simulink model "PhaseEquivalentFOCModel"  (R2020b)
settings: Solver=VariableStepAuto  StartTime=0.0  StopTime=10.0  RelTol=1e-3
libraries: ee_lib x7, nesl_utility x7, mcbcontrolslib x2, eeTransforms x1, eePmsmCurrentController x1, powerlib_meascontrol x1, eeVelocityController x1
settings Model: Creator=trgre  LastModifiedBy=trgre

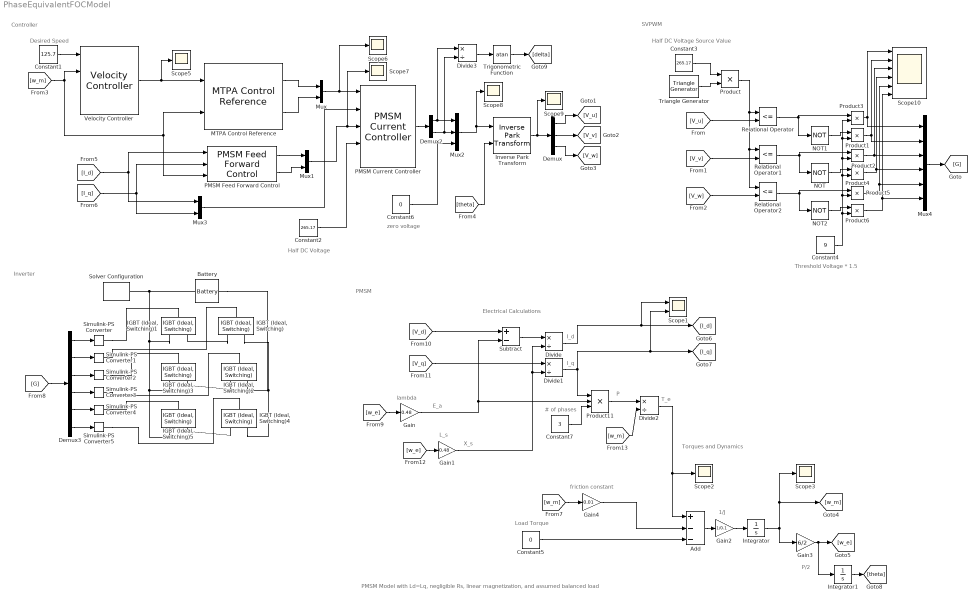
== system PhaseEquivalentFOCModel ==
  note: Load Torque
  note: friction constant
  note: Inverter
  note: PMSM
  note: P/2
  note: 1/J
  note: lambda
  note: Torques and Dynamics
  note: Electrical Calculations
  note: T_e
  note: # of phases
  note: P
  note: PMSM Model with Ld=Lq, negligible Rs, linear magnetization, and assumed balanced load
  note: I_q
  note: I_d
  note: X_s
  note: L_s
  note: E_a
  note: Controller
  note: SVPWM
  note: Desired Speed
  note: Half DC Voltage
  note: zero voltage
  note: Threshold Voltage * 1.5
  note: Half DC Voltage Source Value
  Add : Sum  Inputs=+--
  Battery : ee_lib/Sources/Battery  Vnom=530.35 V  prm_dir=1  R1_dis=2 Ohm  R1_ch=2 Ohm  R1=0.01 Ohm  prm_AH=1  AH=50 hr*A  V1=11.5 V  AH1=25 hr*A  prm_R2=1  R2=2000 Ohm  prm_dyn=1  Rp1=0.005 Ohm  tau1=30 s  Rp2=0.005 Ohm  tau2=30 s  Rp3=0.005 Ohm  tau3=30 s  Rp4=0.005 Ohm  tau4=30 s  Rp5=0.005 Ohm  tau5=30 s  prm_fade=1  N_fade=100  AH_fade=45 hr*A  R1_fade=2.02 Ohm  R1_ch_fade=2.02 Ohm  V1_fade=10.35 V  i_specify=off  i_priority=None  i=0 A  i_nominal_specify=off  i_nominal_unit=A  i_nominal_value=1  v_specify=off  v_priority=None  v=0 V  v_nominal_specify=off  v_nominal_unit=V  v_nominal_value=1  charge_specify=off  charge_priority=High  charge=50 hr*A  charge_nominal_specify=off  charge_nominal_unit=hr*A  charge_nominal_value=1  num_cycles_specify=off  num_cycles_priority=High  num_cycles=0  num_cycles_nominal_specify=off  num_cycles_nominal_unit=1  num_cycles_nominal_value=1  thermal_mass=30000 J/K  Tmeas=298.15 K  Vnom_T2=12 V  R1_T2=2.2 Ohm  R1_T2_dis=2.2 Ohm  R1_T2_ch=2.2 Ohm  V1_T2=11.4 V  R2_T2=2200 Ohm  Rp1_T2=0.005 Ohm  tau1_T2=30 s  Rp2_T2=0.005 Ohm  tau2_T2=30 s  Rp3_T2=0.005 Ohm  tau3_T2=30 s  Rp4_T2=0.005 Ohm  tau4_T2=30 s  Rp5_T2=0.005 Ohm  tau5_T2=30 s  Tmeas2=273.15 K  temperature_specify=off  temperature_priority=High  temperature=298.15 K  temperature_nominal_specify=off  temperature_nominal_unit=K  temperature_nominal_value=1
  Constant1 : Constant  Value=125.7
  Constant2 : Constant  Value=265.17
  Constant3 : Constant  Value=265.17
  Constant4 : Constant  Value=9
  Constant5 : Constant  Value=0
  Constant6 : Constant  Value=0
  Constant7 : Constant  Value=3
  Demux : Demux  Outputs=3
  Demux2 : Demux  Outputs=2
  Demux3 : Demux  Outputs=6
  Divide{,1..3} (4 alike) : Product  Inputs=*/
  Gain : Gain  Gain=0.48
  Gain1 : Gain  Gain=0.48
  Gain2 : Gain  Gain=1/0.1
  Gain3 : Gain  Gain=6/2
  Gain4 : Gain  Gain=0.01
  IGBT (Ideal, Switching){,1..5} (6 alike) : ee_lib/Semiconductors & Converters/IGBT (Ideal, Switching)  Vf=0.8 V  Ron=0.001 Ohm  Goff=1e-5 1/Ohm  Vth=6 V  diode_param=2  diode_Vf=0.8 V  diode_Ron=0.001 Ohm  diode_Goff=1e-5 1/Ohm  diode_C=50e-9 F  diode_iRM=-235 A  diode_iF=300 A  diode_idot=-50 A/us  diode_trr_param=1  diode_trr_factor=3  diode_trr=15 us  diode_Qrr=1500 s*uA  thermal_loss_option=ee.enum.converters.thermalLossOption.constantvalues  Von_data=[0, .1, .6, .8, 1, 1.3, 1.6, 2, 2.4; 0, .1, .7, 1, 1.2, 1.5, 1.9, 2.4, 2.8] V  Eon_data=[0, .0024, .024, .12, .2, .48, 1.04, 2.16, 3.24; 0, .003, .03, .15, .25, .6, 1.3, 2.7, 4.05] * 1e-3 J  Eoff_data=[0, .0007, .0066, .033, .066, .17, .33, .83, 1.5; 0, .001, .01, .05, .1, .25, .5, 1.2, 2.2] * 1e-3 J  Tj=[298.15, 398.15] K  Iout_data=[0, .1, 1, 5, 10, 20, 40, 70, 100] A  Eon_scalar=22.86e-3 J  Eoff_scalar=17.14e-3 J  Voff=300 V  Iout_scalar=600 A  diodeModelType=ee.enum.converters.diodeModelType.pwl  diode_IfMat=[.07, .12, .19, 1.75, 4.24, 7.32, 11.2; .16, .3, .72, 2.14, 4.02, 6.35, 9.12] A  diode_TjVec=[25, 125] degC  diode_VfVec=[.5, .7, .9, 1.3, 1.7, 2.1, 2.5] V  thermal_network_parameterization=ee.enum.thermalNetworkTopology.external  Rth=[.08, .5] K/W  Rth_Foster=[.08, .14, .22, .16] K/W  thermal_mass_parameterization=ee.enum.thermalNetwork.timeconstant  thermal_mass=[.01, .5] J/K  thermal_mass_Foster=[.001, .005, .05, .5] J/K  thermal_time_constant=[.001, .2] s  thermal_time_constant_Foster=[7e-05, .0007, .01, .08] s  thermal_mass_initial_temperatures=[25, 25] degC  junction_thermal_mass=0.01 J/K  Tau=1e-4 s  vT_specify=off  vT_priority=None  vT=0 V  vT_nominal_specify=off  vT_nominal_unit=V  vT_nominal_value=1  Qj_specify=off  Qj_priority=None  Qj=0 W  Qj_nominal_specify=off  Qj_nominal_unit=W  Qj_nominal_value=1  junction_temperature_specify=off  junction_temperature_priority=None  junction_temperature=25 degC  junction_temperature_nominal_specify=off  junction_temperature_nominal_unit=degC  junction_temperature_nominal_value=1
  Integrator : Integrator  InitialCondition=125.7
  Integrator1 : Integrator
  Inverse Park Transform : eeTransforms/Inverse Park Transform  AxisAlignment=Q-axis  PowerInvariant=off
  MTPA Control Reference : mcbcontrolslib/MTPA Control Reference  LabelModeActiveChoice=Surface PMSM  VariantSelect=Surface PMSM  polePairs=3  Rs=0.36  Ld=0.00137  Lq=0.4e-3  FluxPM=0.48  I_sat=7.1  V_dc=24  Units=SI Units  N_base=1200  I_base=19.3  T_base=1  N_base_disp=3182
      settings: SourceProductBaseCode=MT
  Mux : Mux  Inputs=2
  Mux1 : Mux  Inputs=2
  Mux2 : Mux  Inputs=3
  Mux3 : Mux  Inputs=2
  Mux4 : Mux  Inputs=6
  NOT : Logic  Operator=NOT  IconShape=distinctive  AllPortsSameDT=off  OutDataTypeStr=boolean
  NOT1 : Logic  Operator=NOT  IconShape=distinctive  AllPortsSameDT=off  OutDataTypeStr=boolean
  NOT2 : Logic  Operator=NOT  IconShape=distinctive  AllPortsSameDT=off  OutDataTypeStr=boolean
  PMSM Current Controller : eePmsmCurrentController/PMSM Current Controller  Kp_id=1  Ki_id=100  Kaw_id=1  Kp_iq=1  Ki_iq=100  Kaw_iq=1  Ts=-1  Tsd=0.001  AxisPrio=Q-axis  ActZC=off  ActFF=on
      settings: SourceProductBaseCode=PS
  PMSM Feed Forward Control : mcbcontrolslib/PMSM Feed Forward Control  polePairs=3  Ld=0.00137  Lq=0.00137  FluxPM=0.48  V_dc=24/sqrt(3)  Units=SI Units  V_base=24/sqrt(3)  I_base=19.3  N_base=4107
      settings: SourceProductBaseCode=MT
  Product{,1..6} (7 alike) : Product
  Product11 : Product  Inputs=3
  Relational Operator : RelationalOperator  Operator=<=  OutDataTypeStr=boolean  RndMeth=Simplest
  Relational Operator1 : RelationalOperator  Operator=<=  OutDataTypeStr=boolean  RndMeth=Simplest
  Relational Operator2 : RelationalOperator  Operator=<=  OutDataTypeStr=boolean  RndMeth=Simplest
  Scope1 : Scope  NumInputPorts=2
  Scope10 : Scope  NumInputPorts=6
  Scope{2..3,5..9} (7 alike) : Scope
  Simulink-PS Converter{,1..5} (6 alike) : nesl_utility/Simulink-PS Converter  PhysicalDomain=network_engine_domain  SubClassName=ps_input  LeftPortType=input  RightPortType=output  PseudoPeriodic=off  Frequencies=[]  NoiseDistribution=none  NoiseParameters=[]  Unit=1  AffineConversion=off  FilteringAndDerivatives=provide  SimscapeFilterOrder=1  InputFilterTimeConstant=0.001  UdotUserProvided=0
  Solver Configuration : nesl_utility/Solver Configuration  PhysicalDomain=network_engine_domain  SubClassName=solver  LeftPortType=input  RightPortType=generic  Tones=[]  Harmonics=[]  SimulateNoise=off  Profile=off  UseLocalSampling=off  EnableSwitchedLinearOptims=on  FrequencyDomain=off  UseCCode=off  RelTol=0.001  AbsTol=1e-06  MinStep=1e-09  ToWorkspace=off  RevertToSquareIcSolve=off  NumHomotopyIterations=100  PhasorMode=off  PhasorModeNumHarmonics=1  DoDC=off  ResidualTolerance=1e-09  UseLocalSolver=off  LocalSolverChoice=NE_BACKWARD_EULER_ADVANCER  LocalSolverSampleTime=0.001  DoFixedCost=off  MaxNonlinIter=3  MaxModeIter=2  ComputeImpulses=off  ImpulseIterations=2  LinearAlgebra=auto  EquationFormulation=NE_TIME_EF  DelaysMemoryBudget=1024  AutomaticFiltering=on  FilteringTimeConstant=0.001  PartitionStorageMethod=AS_NEEDED  PartitionMemoryBudget=1024  PartitionMethod=ROBUST
  Subtract : Sum  Inputs=+-
  Triangle Generator : powerlib_meascontrol/Pulse & Signal Generators/Triangle Generator  Freq=10e3  Phase=90  Ts=0
  Trigonometric Function : Trigonometry  Operator=atan
  Velocity Controller : eeVelocityController/Velocity Controller  CtrlType=PI control  Kp_w=1  Ki_w=1  Kv_w=1  Kaw_w=1  Ts=-1  Tsd=0.001  ActZC=off
      settings: SourceProductBaseCode=PS
  wires:
  Relational Operator2/1 -> NOT2/1, Product5/1
  Relational Operator/1 -> NOT1/1, Product3/1
  Relational Operator1/1 -> NOT/1, Product2/1
  Inverse Park Transform/1 -> Scope9/1, Demux/1
  Constant3/1 -> Product/1
  Triangle Generator/1 -> Product/2
  Product/1 -> Relational Operator/1, Relational Operator1/1, Relational Operator2/1
  Product4/1 -> Mux4/4, Scope10/4
  Product5/1 -> Mux4/5, Scope10/5
  Product6/1 -> Mux4/6, Scope10/6
  Product2/1 -> Mux4/3, Scope10/3
  Product1/1 -> Mux4/2, Scope10/2
  Product3/1 -> Mux4/1, Scope10/1
  NOT1/1 -> Product1/1
  NOT/1 -> Product4/1
  NOT2/1 -> Product6/1
  Constant4/1 -> Product6/2, Product5/2, Product4/2, Product2/2, Product1/2, Product3/2
  MTPA Control Reference/1 -> Mux/1
  MTPA Control Reference/2 -> Mux/2
  Mux/1 -> Scope6/1, PMSM Current Controller/1
  Velocity Controller/1 -> Scope5/1, MTPA Control Reference/1
  PMSM Feed Forward Control/1 -> Mux1/1
  PMSM Feed Forward Control/2 -> Mux1/2
  Mux1/1 -> Scope7/1, PMSM Current Controller/3
  Constant1/1 -> Velocity Controller/1
  Constant2/1 -> PMSM Current Controller/4
  PMSM Current Controller/1 -> Demux2/1
  Demux2/2 -> Divide3/2, Mux2/2
  Mux2/1 -> Scope8/1, Inverse Park Transform/1
  Constant6/1 -> Mux2/3
  Mux3/1 -> PMSM Current Controller/2
  [V_u] -> Relational Operator/2
  [V_v] -> Relational Operator1/2
  [V_w] -> Relational Operator2/2
  Mux4/1 -> [G]
  [w_m] -> PMSM Feed Forward Control/3, MTPA Control Reference/2, Velocity Controller/2
  Demux/1 -> [V_u]
  Demux/2 -> [V_v]
  Demux/3 -> [V_w]
  [G] -> Demux3/1
  [V_d] -> Subtract/1
  Gain/1 -> Subtract/2, Product11/2
  Subtract/1 -> Divide/1
  Gain1/1 -> Divide1/2, Divide/2
  [V_q] -> Divide1/1
  Divide1/1 -> Product11/1, Scope1/2, [I_q]
  Constant7/1 -> Product11/3
  Product11/1 -> Divide2/1
  [w_m] -> Divide2/2
  Divide2/1 -> Scope2/1, Add/1
  [w_e] -> Gain/1
  [w_e] -> Gain1/1
  Add/1 -> Gain2/1
  Gain2/1 -> Integrator/1
  Integrator/1 -> Gain3/1, Scope3/1, [w_m]
  Gain3/1 -> Integrator1/1, [w_e]
  [theta] -> Inverse Park Transform/2
  Divide/1 -> Scope1/1, [I_d]
  [I_d] -> Mux3/1, PMSM Feed Forward Control/1
  [I_q] -> Mux3/2, PMSM Feed Forward Control/2
  [w_m] -> Gain4/1
  Gain4/1 -> Add/2
  Constant5/1 -> Add/3
  Integrator1/1 -> [theta]
  Divide3/1 -> Trigonometric Function/1
  Demux2/1 -> Divide3/1, Mux2/1
  Trigonometric Function/1 -> [delta]
  Demux3/1 -> Simulink-PS Converter/1
  Demux3/2 -> Simulink-PS Converter1/1
  Demux3/3 -> Simulink-PS Converter2/1
  Demux3/4 -> Simulink-PS Converter3/1
  Demux3/5 -> Simulink-PS Converter4/1
  Demux3/6 -> Simulink-PS Converter5/1
  connections:
  "IGBT (Ideal, Switching)3"/RConn2 -- "IGBT (Ideal, Switching)5"/RConn2 -- "IGBT (Ideal, Switching)1"/RConn2 -- Battery/LConn1 -- Solver Configuration/RConn1
  "IGBT (Ideal, Switching)2"/RConn1 -- Battery/RConn1 -- "IGBT (Ideal, Switching)"/RConn1 -- "IGBT (Ideal, Switching)4"/RConn1
  "IGBT (Ideal, Switching)"/RConn2 -- "IGBT (Ideal, Switching)1"/RConn1
  "IGBT (Ideal, Switching)4"/RConn2 -- "IGBT (Ideal, Switching)5"/RConn1
  "IGBT (Ideal, Switching)2"/RConn2 -- "IGBT (Ideal, Switching)3"/RConn1
  Simulink-PS Converter/RConn1 -- "IGBT (Ideal, Switching)1"/LConn1
  Simulink-PS Converter1/RConn1 -- "IGBT (Ideal, Switching)"/LConn1
  Simulink-PS Converter2/RConn1 -- "IGBT (Ideal, Switching)3"/LConn1
  Simulink-PS Converter3/RConn1 -- "IGBT (Ideal, Switching)2"/LConn1
  Simulink-PS Converter4/RConn1 -- "IGBT (Ideal, Switching)5"/LConn1
  Simulink-PS Converter5/RConn1 -- "IGBT (Ideal, Switching)4"/LConn1
